simulink model "DC_correction_testing"  (R2024b)
settings: Solver=FixedStepAuto  StartTime=0.0  StopTime=inf  FixedStep=1/Param.Fs  RelTol=1e-3
undefined symbols (not defined in the file): Fs, ip, Param, usb
libraries: plutoradiolib x2, dspsigops x2, commfilt2 x2, commrfcorlib x1, commsink2 x1, commsync2 x1
settings Model: Creator=rober  LastModifiedBy=rober

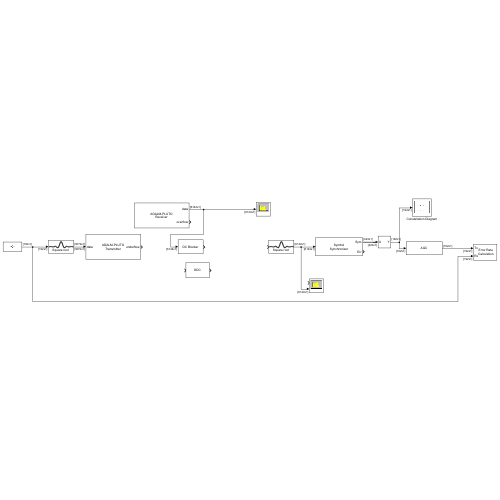
[thumbnail: Simulink's stored preview of the top-level diagram]
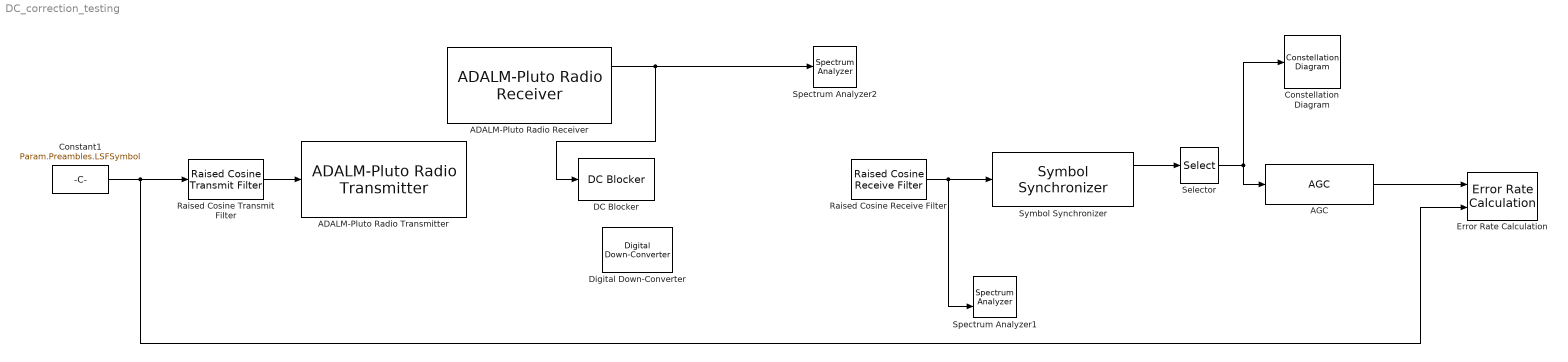
== system DC_correction_testing ==
  ADALM-Pluto Radio Receiver : plutoradiolib/ADALM-Pluto Radio Receiver  RadioID=usb:0  uri=ip:10.0.0.200  CenterFrequencySource=Dialog  CenterFrequency=Param.PlutoCenterFrequency  GainSource=AGC Slow Attack  GainSourceBlock=AGC Slow Attack  Gain=10  ChannelMapping=1  BasebandSampleRate=Param.Fs*2  OutputDataType=double  SamplesPerFrame=Param.PlutoFrameLength*2  OverflowOutputPort=on  EnableBurstMode=off  NumFramesInBurst=1  ShowAdvancedProperties=off  UseCustomFilter=off  filtPathRates=[737280000 11520000 3840000 1920000 960000 240000]  filtCoefficients=[-192 82 85 -215 228 -102 -110 290 -318 145 160 -426 471 -215 -238 633 -697 318 349 -923 1009 -457 -498 1309 -1423 640 693 -1812 1959 -876 -945 2458 -2647 1180 1268 -3290 3534 -1572 -1688 4375 -4698 2091 2247 -5836 6284 -2807 -3031 7918 -8588 3870 4225 -11182 12324 -5662 -6330 17255 -19735 9507 11312 -33568 43355 -25227 -42139 305542 305542 -42139 -25227 43355 -33568 11312 9507 -19735 17255 -6330 -5662 12324 -11182 4225 3870 -8588 7918 -3031 -2807 6284 -5836 2247 2091 -4698 4375 -1688 -1572 3534 -3290 1268 1180 -2647 2458 -945 -876 1959 -1812 693 640 -1423 1309 -498 -457 1009 -923 349 318 -697 633 -238 -215 471 -426 160 145 -318 290 -110 -102 228 -215 85 82 -192]  filtCoefficientSize=128  filtDecimInterpFactor=4  filtGain=-12  filtRFBandwidth=18000000  filterConfigStruct=struct()  EnableQuadratureCorrection=on  EnableRFDCCorrection=on  EnableBasebandDCCorrection=on  FrequencyCorrection=0  OverrideSampleTime=off  SampleTime=0.02  DataTimeout=Inf  ENSMPinControlMode=None  BISTLoopbackMode=Disabled  BISTToneInject=Disabled  BISTSignalGen=PRBS  BISTToneFreq=Fs/32  BISTToneLevel=0
  ADALM-Pluto Radio Transmitter : plutoradiolib/ADALM-Pluto Radio Transmitter  RadioID=usb:0  uri=ip:10.0.0.200  CenterFrequencySource=Dialog  CenterFrequency=Param.PlutoCenterFrequency+10e3  GainSource=Dialog  Gain=0  ChannelMapping=1  BasebandSampleRate=Param.Fs  UnderflowOutputPort=on  ShowAdvancedProperties=off  UseCustomFilter=off  filtPathRates=[737280000 11520000 3840000 1920000 960000 240000]  filtCoefficients=[-192 82 85 -215 228 -102 -110 290 -318 145 160 -426 471 -215 -238 633 -697 318 349 -923 1009 -457 -498 1309 -1423 640 693 -1812 1959 -876 -945 2458 -2647 1180 1268 -3290 3534 -1572 -1688 4375 -4698 2091 2247 -5836 6284 -2807 -3031 7918 -8588 3870 4225 -11182 12324 -5662 -6330 17255 -19735 9507 11312 -33568 43355 -25227 -42139 305542 305542 -42139 -25227 43355 -33568 11312 9507 -19735 17255 -6330 -5662 12324 -11182 4225 3870 -8588 7918 -3031 -2807 6284 -5836 2247 2091 -4698 4375 -1688 -1572 3534 -3290 1268 1180 -2647 2458 -945 -876 1959 -1812 693 640 -1423 1309 -498 -457 1009 -923 349 318 -697 633 -238 -215 471 -426 160 145 -318 290 -110 -102 228 -215 85 82 -192]  filtCoefficientSize=128  filtDecimInterpFactor=4  filtGain=-12  filtRFBandwidth=18000000  filterConfigStruct=struct()  DataSourceSelect=Input Port  DDSTone1Freq=5e3  DDSTone2Freq=10e3  DDSTone1Scale=0.5  DDSTone2Scale=0.25  DataTimeout=Inf  FrequencyCorrection=0  ENSMPinControlMode=None  BISTLoopbackMode=Disabled  BISTToneInject=Disabled  BISTSignalGen=PRBS  BISTToneFreq=Fs/32  BISTToneLevel=0
  AGC : commrfcorlib/AGC  LegacyMode=off  DetectorMethod=Rectifier  LoopMethod=Linear  UpdatePeriod=100  StepSize=0.1  AdaptationStepSize=0.01  DesiredOutputPower=1  AveragingLength=100  MaximumGain=30  MaxPowerGain=60  GainOutputPort=off  InputPowerOutputPort=off  SimulateUsing=Interpreted execution
  Constant1 : Constant  Value=Param.Preambles.LSFSymbol  VectorParams1D=off
  Constellation Diagram : ConstellationDiagram  WindowPosition=[328.000000,69.000000,600.000000,600.000000,]  Visible=on  ScopeFrameLocation=window
  DC Blocker : dspsigops/DC Blocker  Algorithm=IIR  NormalizedBandwidth=0.001  Length=8  Order=6  SimulateUsing=Code generation
      settings: LibrarySourceBlock=commhdlfilt/DC Blocker
  Digital Down-Converter : dspsigops/Digital Down-Converter  DecimationFactor=100  MinimumOrderDesign=on  NumCICSections=3  ThirdFilterOrder=10  StopbandFrequencySource=Auto  Oscillator=Sine wave  CenterFrequency=0.9333  SecondFilterOrder=12  Bandwidth=0.0133  StopbandFrequency=0.01  PassbandRipple=0.1  StopbandAttenuation=60  NumAccumulatorBits=16  NumQuantizedAccumulatorBits=12  Dither=on  NumDitherBits=4  SampleRateMode=Use normalized frequency (0 to 1)  SampleRate=30e6  SimulateUsing=Interpreted execution  outputMin=[]  outputMax=[]
  Error Rate Calculation : commsink2/Error Rate Calculation  N=0  st_delay=0  cp_mode=Entire frame  subframe=[]  PMode=Workspace  WsName=ErrorVec  RsMode2=off  stop=off  numErr=100  maxBits=1e6
  Raised Cosine Receive Filter : commfilt2/Raised Cosine Receive Filter  filtType=Square root  R=0.5  filtSpan=Param.RaisedCosineFilterSpan  N=Param.Interpolation  downFactor=1  downOffset=0  filterGain=1  InputProcessing=Columns as channels (frame based)  RateOptions=Enforce single-rate processing  framing=Mute  checkCoeff=off  variableName=rcRxFilt  currentFiltSpan=10  D=5  inputOffset=0  sampMode=Mute  saveAsFlag=0  rateMode=Downsampling  checkGain=Normalized  launchFVT=on  roundingMode=Floor  overflowMode=off  coeffDataTypeStr=Inherit: Same word length as input  coeffMin=[]  coeffMax=[]  coeffLastDataTypeStr=Inherit: Same word length as input  accumDataTypeStr=Inherit: Same as product output  accumLastDataTypeStr=Inherit: Same as product output  outputDataTypeStr=Inherit: Same as accumulator  outputMin=[]  outputMax=[]  outputLastDataTypeStr=Inherit: Same as accumulator
  Raised Cosine Transmit Filter : commfilt2/Raised Cosine Transmit Filter  filtType=Square root  R=0.5  filtSpan=Param.RaisedCosineFilterSpan  N=Param.Interpolation  filterGain=1  InputProcessing=Columns as channels (frame based)  RateOptions=Enforce single-rate processing  framing=Mute  checkCoeff=off  variableName=rcTxFilt  checkGain=Normalized  sampMode=Mute  saveAsFlag=0  currentFiltSpan=10  D=(10)/2  launchFVT=on  roundingMode=Floor  overflowMode=off  coeffDataTypeStr=Inherit: Same word length as input  coeffMin=[]  coeffMax=[]  coeffLastDataTypeStr=Inherit: Same word length as input  outputDataTypeStr=Inherit: Same as accumulator  outputMin=[]  outputMax=[]  outputLastDataTypeStr=Inherit: Same as accumulator
  Selector : Selector  IndexOptions=Index vector (dialog)  Indices=[1:192]  OutputSizes=1
  Spectrum Analyzer1 : SpectrumAnalyzer  NumInputPorts=2  WindowPosition=[-25.000000,77.000000,800.000000,576.000000,]  Visible=on  ScopeFrameLocation=window  WindowInvariantSamplesPerUpdate=on  Span=144000  StartFrequency=-72000  StopFrequency=72000  YLimits=[-185.5160190185582,72.18608117144183]
      settings: OpenAtSimulationStart=off
  Spectrum Analyzer2 : SpectrumAnalyzer  WindowPosition=[271.000000,80.000000,800.000000,576.000000,]  Visible=on  ScopeFrameLocation=window  WindowInvariantSamplesPerUpdate=on  Span=442368000  StartFrequency=-221184000  StopFrequency=221184000  YLimits=[-43.85961656823777,8.715932461762229]
      settings: OpenAtSimulationStart=off
  Symbol Synchronizer : commsync2/Symbol Synchronizer  Modulation=PAM/PSK/QAM  TimingErrorDetector=Gardner (non-data-aided)  SamplesPerSymbol=16  DampingFactor=1  NormalizedLoopBandwidth=0.01  DetectorGain=2.7  TimingErrorOutputPort=on  SimulateUsing=Code generation
  wires:
  Raised Cosine Transmit Filter/1 -> ADALM-Pluto Radio Transmitter/1
  Constant1/1 -> Raised Cosine Transmit Filter/1, Error Rate Calculation/2
  Raised Cosine Receive Filter/1 -> Spectrum Analyzer1/2, Symbol Synchronizer/1
  Symbol Synchronizer/1 -> Selector/1
  Selector/1 -> AGC/1, Constellation Diagram/1
  AGC/1 -> Error Rate Calculation/1
  ADALM-Pluto Radio Receiver/1 -> DC Blocker/1, Spectrum Analyzer2/1
